simulink model "Intergration_simu"  (R2018b)
settings: Solver=FixedStepDiscrete  StartTime=0.0  StopTime=14  FixedStep=0.005  RelTol=1e-3
PostLoadFcn:
  | if any(exist('dsrtsu_mdlpostloadfcn', 'file') ~= 0), dsrtsu_mdlpostloadfcn('Execute', bdroot); end
values from neighbouring files (symbols this model uses):
  P_x165_On = 1.0    [CAN_Tx.sldd]
  P_x242_On = 1.0    [CAN_Tx.sldd]
  P_x246_On = 1.0    [CAN_Tx.sldd]
libraries: rtican x112, simulink x59
(part 29 of 31)

== system Intergration_simu/Radar410_RX/Subsystem41/Subsystem21 ==
  In1 : Inport
  Bus Creator : BusCreator  Inputs=20  OutDataTypeStr=Bus: Obj_Data  NonVirtualBus=on
      settings: InheritFromInputs=off
  Bus Selector : BusSelector  OutputSignals=FRS_P1_19_Msg_CheckSum,FRS_P1_19_Msg_AliveCounter,FRS_P1_19_Obj_ExstProb,FRS_P1_19_Obj_XVelRel_Stdev,FRS_P1_19_Obj_XAccRel,FRS_P1_19_Obj_ObstacleProb,FRS_P1_19_Obj_MotionPattern,FRS_P1_19_Obj_YPos_Stdev,FRS_P1_19_Obj_ValidFlag,FRS_P1_19_Obj_XPos_Stdev,FRS_P1_19_Obj_UpdateFlag,FRS_P1_19_Obj_ID,FRS_P2_19_Msg_CheckSum,FRS_P2_19_Msg_AliveCounter,FRS_P2_19_Obj_MeasFlag,FRS_P2_19_Obj_YVelRel,FRS_P2_19_Obj_Type,FRS_P2_19_Obj_XPos,FRS_P2_19_Obj_YPos,FRS_P2_19_Obj_XVelRel
  Data Type Conversion{,1..19} (20 alike) : DataTypeConversion  OutDataTypeStr=single
  Out1 : Outport  OutDataTypeStr=Bus: Obj_Data
  wires:
  Data Type Conversion19/1 -> Bus Creator/20
  Data Type Conversion14/1 -> Bus Creator/15
  Data Type Conversion8/1 -> Bus Creator/9
  Data Type Conversion7/1 -> Bus Creator/8
  Data Type Conversion3/1 -> Bus Creator/4
  Data Type Conversion4/1 -> Bus Creator/5
  Data Type Conversion1/1 -> Bus Creator/2
  Data Type Conversion13/1 -> Bus Creator/14
  Data Type Conversion2/1 -> Bus Creator/3
  Data Type Conversion/1 -> Bus Creator/1
  Bus Creator/1 -> Out1/1
  In1/1 -> Bus Selector/1
  Bus Selector/20 -> Data Type Conversion19/1  "<FRS_P2_19_Obj_XVelRel>"
  Bus Selector/18 -> Data Type Conversion17/1  "<FRS_P2_19_Obj_XPos>"
  Bus Selector/19 -> Data Type Conversion18/1  "<FRS_P2_19_Obj_YPos>"
  Bus Selector/14 -> Data Type Conversion13/1  "<FRS_P2_19_Msg_AliveCounter>"
  Data Type Conversion10/1 -> Bus Creator/11
  Bus Selector/10 -> Data Type Conversion9/1  "<FRS_P1_19_Obj_XPos_Stdev>"
  Bus Selector/17 -> Data Type Conversion16/1  "<FRS_P2_19_Obj_Type>"
  Bus Selector/9 -> Data Type Conversion8/1  "<FRS_P1_19_Obj_ValidFlag>"
  Data Type Conversion16/1 -> Bus Creator/17
  Bus Selector/12 -> Data Type Conversion11/1  "<FRS_P1_19_Obj_ID>"
  Data Type Conversion6/1 -> Bus Creator/7
  Bus Selector/16 -> Data Type Conversion15/1  "<FRS_P2_19_Obj_YVelRel>"
  Data Type Conversion17/1 -> Bus Creator/18
  Bus Selector/11 -> Data Type Conversion10/1  "<FRS_P1_19_Obj_UpdateFlag>"
  Data Type Conversion18/1 -> Bus Creator/19
  Bus Selector/6 -> Data Type Conversion5/1  "<FRS_P1_19_Obj_ObstacleProb>"
  Data Type Conversion9/1 -> Bus Creator/10
  Bus Selector/7 -> Data Type Conversion6/1  "<FRS_P1_19_Obj_MotionPattern>"
  Bus Selector/4 -> Data Type Conversion3/1  "<FRS_P1_19_Obj_XVelRel_Stdev>"
  Data Type Conversion5/1 -> Bus Creator/6
  Data Type Conversion11/1 -> Bus Creator/12
  Bus Selector/2 -> Data Type Conversion1/1  "<FRS_P1_19_Msg_AliveCounter>"
  Bus Selector/13 -> Data Type Conversion12/1  "<FRS_P2_19_Msg_CheckSum>"
  Bus Selector/3 -> Data Type Conversion2/1  "<FRS_P1_19_Obj_ExstProb>"
  Bus Selector/15 -> Data Type Conversion14/1  "<FRS_P2_19_Obj_MeasFlag>"
  Bus Selector/1 -> Data Type Conversion/1  "<FRS_P1_19_Msg_CheckSum>"
  Data Type Conversion15/1 -> Bus Creator/16
  Bus Selector/8 -> Data Type Conversion7/1  "<FRS_P1_19_Obj_YPos_Stdev>"
  Bus Selector/5 -> Data Type Conversion4/1  "<FRS_P1_19_Obj_XAccRel>"
  Data Type Conversion12/1 -> Bus Creator/13

== system Intergration_simu/Radar410_RX/Subsystem41/Subsystem22 ==
  In1 : Inport
  Bus Creator : BusCreator  Inputs=20  OutDataTypeStr=Bus: Obj_Data  NonVirtualBus=on
      settings: InheritFromInputs=off
  Bus Selector : BusSelector  OutputSignals=FRS_P1_20_Msg_CheckSum,FRS_P1_20_Msg_AliveCounter,FRS_P1_20_Obj_ExstProb,FRS_P1_20_Obj_XVelRel_Stdev,FRS_P1_20_Obj_XAccRel,FRS_P1_20_Obj_ObstacleProb,FRS_P1_20_Obj_MotionPattern,FRS_P1_20_Obj_YPos_Stdev,FRS_P1_20_Obj_ValidFlag,FRS_P1_20_Obj_XPos_Stdev,FRS_P1_20_Obj_UpdateFlag,FRS_P1_20_Obj_ID,FRS_P2_20_Msg_CheckSum,FRS_P2_20_Msg_AliveCounter,FRS_P2_20_Obj_MeasFlag,FRS_P2_20_Obj_YVelRel,FRS_P2_20_Obj_Type,FRS_P2_20_Obj_XPos,FRS_P2_20_Obj_YPos,FRS_P2_20_Obj_XVelRel
  Data Type Conversion{,1..19} (20 alike) : DataTypeConversion  OutDataTypeStr=single
  Out1 : Outport  OutDataTypeStr=Bus: Obj_Data
  wires:
  Data Type Conversion19/1 -> Bus Creator/20
  Data Type Conversion14/1 -> Bus Creator/15
  Data Type Conversion8/1 -> Bus Creator/9
  Data Type Conversion7/1 -> Bus Creator/8
  Data Type Conversion3/1 -> Bus Creator/4
  Data Type Conversion4/1 -> Bus Creator/5
  Data Type Conversion1/1 -> Bus Creator/2
  Data Type Conversion13/1 -> Bus Creator/14
  Data Type Conversion2/1 -> Bus Creator/3
  Data Type Conversion/1 -> Bus Creator/1
  Bus Creator/1 -> Out1/1
  In1/1 -> Bus Selector/1
  Bus Selector/20 -> Data Type Conversion19/1  "<FRS_P2_20_Obj_XVelRel>"
  Bus Selector/18 -> Data Type Conversion17/1  "<FRS_P2_20_Obj_XPos>"
  Bus Selector/19 -> Data Type Conversion18/1  "<FRS_P2_20_Obj_YPos>"
  Bus Selector/14 -> Data Type Conversion13/1  "<FRS_P2_20_Msg_AliveCounter>"
  Data Type Conversion10/1 -> Bus Creator/11
  Bus Selector/10 -> Data Type Conversion9/1  "<FRS_P1_20_Obj_XPos_Stdev>"
  Bus Selector/17 -> Data Type Conversion16/1  "<FRS_P2_20_Obj_Type>"
  Bus Selector/9 -> Data Type Conversion8/1  "<FRS_P1_20_Obj_ValidFlag>"
  Data Type Conversion16/1 -> Bus Creator/17
  Bus Selector/12 -> Data Type Conversion11/1  "<FRS_P1_20_Obj_ID>"
  Data Type Conversion6/1 -> Bus Creator/7
  Bus Selector/16 -> Data Type Conversion15/1  "<FRS_P2_20_Obj_YVelRel>"
  Data Type Conversion17/1 -> Bus Creator/18
  Bus Selector/11 -> Data Type Conversion10/1  "<FRS_P1_20_Obj_UpdateFlag>"
  Data Type Conversion18/1 -> Bus Creator/19
  Bus Selector/6 -> Data Type Conversion5/1  "<FRS_P1_20_Obj_ObstacleProb>"
  Data Type Conversion9/1 -> Bus Creator/10
  Bus Selector/7 -> Data Type Conversion6/1  "<FRS_P1_20_Obj_MotionPattern>"
  Bus Selector/4 -> Data Type Conversion3/1  "<FRS_P1_20_Obj_XVelRel_Stdev>"
  Data Type Conversion5/1 -> Bus Creator/6
  Data Type Conversion11/1 -> Bus Creator/12
  Bus Selector/2 -> Data Type Conversion1/1  "<FRS_P1_20_Msg_AliveCounter>"
  Bus Selector/13 -> Data Type Conversion12/1  "<FRS_P2_20_Msg_CheckSum>"
  Bus Selector/3 -> Data Type Conversion2/1  "<FRS_P1_20_Obj_ExstProb>"
  Bus Selector/15 -> Data Type Conversion14/1  "<FRS_P2_20_Obj_MeasFlag>"
  Bus Selector/1 -> Data Type Conversion/1  "<FRS_P1_20_Msg_CheckSum>"
  Data Type Conversion15/1 -> Bus Creator/16
  Bus Selector/8 -> Data Type Conversion7/1  "<FRS_P1_20_Obj_YPos_Stdev>"
  Bus Selector/5 -> Data Type Conversion4/1  "<FRS_P1_20_Obj_XAccRel>"
  Data Type Conversion12/1 -> Bus Creator/13

== system Intergration_simu/Radar410_RX/Subsystem41/Subsystem23 ==
  In1 : Inport
  Bus Creator : BusCreator  Inputs=20  OutDataTypeStr=Bus: Obj_Data  NonVirtualBus=on
      settings: InheritFromInputs=off
  Bus Selector : BusSelector  OutputSignals=FRS_P1_21_Msg_CheckSum,FRS_P1_21_Msg_AliveCounter,FRS_P1_21_Obj_ExstProb,FRS_P1_21_Obj_XVelRel_Stdev,FRS_P1_21_Obj_XAccRel,FRS_P1_21_Obj_ObstacleProb,FRS_P1_21_Obj_MotionPattern,FRS_P1_21_Obj_YPos_Stdev,FRS_P1_21_Obj_ValidFlag,FRS_P1_21_Obj_XPos_Stdev,FRS_P1_21_Obj_UpdateFlag,FRS_P1_21_Obj_ID,FRS_P2_21_Msg_CheckSum,FRS_P2_21_Msg_AliveCounter,FRS_P2_21_Obj_MeasFlag,FRS_P2_21_Obj_YVelRel,FRS_P2_21_Obj_Type,FRS_P2_21_Obj_XPos,FRS_P2_21_Obj_YPos,FRS_P2_21_Obj_XVelRel
  Data Type Conversion{,1..19} (20 alike) : DataTypeConversion  OutDataTypeStr=single
  Out1 : Outport  OutDataTypeStr=Bus: Obj_Data
  wires:
  Data Type Conversion12/1 -> Bus Creator/13
  Bus Selector/5 -> Data Type Conversion4/1  "<FRS_P1_21_Obj_XAccRel>"
  Bus Selector/8 -> Data Type Conversion7/1  "<FRS_P1_21_Obj_YPos_Stdev>"
  Data Type Conversion15/1 -> Bus Creator/16
  Bus Selector/1 -> Data Type Conversion/1  "<FRS_P1_21_Msg_CheckSum>"
  Bus Selector/15 -> Data Type Conversion14/1  "<FRS_P2_21_Obj_MeasFlag>"
  Bus Selector/3 -> Data Type Conversion2/1  "<FRS_P1_21_Obj_ExstProb>"
  Bus Selector/13 -> Data Type Conversion12/1  "<FRS_P2_21_Msg_CheckSum>"
  Bus Selector/2 -> Data Type Conversion1/1  "<FRS_P1_21_Msg_AliveCounter>"
  Data Type Conversion11/1 -> Bus Creator/12
  Data Type Conversion5/1 -> Bus Creator/6
  Bus Selector/4 -> Data Type Conversion3/1  "<FRS_P1_21_Obj_XVelRel_Stdev>"
  Bus Selector/7 -> Data Type Conversion6/1  "<FRS_P1_21_Obj_MotionPattern>"
  Data Type Conversion9/1 -> Bus Creator/10
  Bus Selector/6 -> Data Type Conversion5/1  "<FRS_P1_21_Obj_ObstacleProb>"
  Data Type Conversion18/1 -> Bus Creator/19
  Bus Selector/11 -> Data Type Conversion10/1  "<FRS_P1_21_Obj_UpdateFlag>"
  Data Type Conversion17/1 -> Bus Creator/18
  Bus Selector/16 -> Data Type Conversion15/1  "<FRS_P2_21_Obj_YVelRel>"
  Data Type Conversion6/1 -> Bus Creator/7
  Bus Selector/12 -> Data Type Conversion11/1  "<FRS_P1_21_Obj_ID>"
  Data Type Conversion16/1 -> Bus Creator/17
  Bus Selector/9 -> Data Type Conversion8/1  "<FRS_P1_21_Obj_ValidFlag>"
  Bus Selector/17 -> Data Type Conversion16/1  "<FRS_P2_21_Obj_Type>"
  Bus Selector/10 -> Data Type Conversion9/1  "<FRS_P1_21_Obj_XPos_Stdev>"
  Data Type Conversion10/1 -> Bus Creator/11
  Bus Selector/14 -> Data Type Conversion13/1  "<FRS_P2_21_Msg_AliveCounter>"
  Bus Selector/19 -> Data Type Conversion18/1  "<FRS_P2_21_Obj_YPos>"
  Bus Selector/18 -> Data Type Conversion17/1  "<FRS_P2_21_Obj_XPos>"
  Bus Selector/20 -> Data Type Conversion19/1  "<FRS_P2_21_Obj_XVelRel>"
  In1/1 -> Bus Selector/1
  Bus Creator/1 -> Out1/1
  Data Type Conversion/1 -> Bus Creator/1
  Data Type Conversion2/1 -> Bus Creator/3
  Data Type Conversion13/1 -> Bus Creator/14
  Data Type Conversion1/1 -> Bus Creator/2
  Data Type Conversion4/1 -> Bus Creator/5
  Data Type Conversion3/1 -> Bus Creator/4
  Data Type Conversion7/1 -> Bus Creator/8
  Data Type Conversion8/1 -> Bus Creator/9
  Data Type Conversion14/1 -> Bus Creator/15
  Data Type Conversion19/1 -> Bus Creator/20

== system Intergration_simu/Radar410_RX/Subsystem41/Subsystem24 ==
  In1 : Inport
  Bus Creator : BusCreator  Inputs=20  OutDataTypeStr=Bus: Obj_Data  NonVirtualBus=on
      settings: InheritFromInputs=off
  Bus Selector : BusSelector  OutputSignals=FRS_P1_24_Msg_CheckSum,FRS_P1_24_Msg_AliveCounter,FRS_P1_24_Obj_ExstProb,FRS_P1_24_Obj_XVelRel_Stdev,FRS_P1_24_Obj_XAccRel,FRS_P1_24_Obj_ObstacleProb,FRS_P1_24_Obj_MotionPattern,FRS_P1_24_Obj_YPos_Stdev,FRS_P1_24_Obj_ValidFlag,FRS_P1_24_Obj_XPos_Stdev,FRS_P1_24_Obj_UpdateFlag,FRS_P1_24_Obj_ID,FRS_P2_24_Msg_CheckSum,FRS_P2_24_Msg_AliveCounter,FRS_P2_24_Obj_MeasFlag,FRS_P2_24_Obj_YVelRel,FRS_P2_24_Obj_Type,FRS_P2_24_Obj_XPos,FRS_P2_24_Obj_YPos,FRS_P2_24_Obj_XVelRel
  Data Type Conversion{,1..19} (20 alike) : DataTypeConversion  OutDataTypeStr=single
  Out1 : Outport  OutDataTypeStr=Bus: Obj_Data
  wires:
  Data Type Conversion12/1 -> Bus Creator/13
  Bus Selector/5 -> Data Type Conversion4/1  "<FRS_P1_24_Obj_XAccRel>"
  Bus Selector/8 -> Data Type Conversion7/1  "<FRS_P1_24_Obj_YPos_Stdev>"
  Data Type Conversion15/1 -> Bus Creator/16
  Bus Selector/1 -> Data Type Conversion/1  "<FRS_P1_24_Msg_CheckSum>"
  Bus Selector/15 -> Data Type Conversion14/1  "<FRS_P2_24_Obj_MeasFlag>"
  Bus Selector/3 -> Data Type Conversion2/1  "<FRS_P1_24_Obj_ExstProb>"
  Bus Selector/13 -> Data Type Conversion12/1  "<FRS_P2_24_Msg_CheckSum>"
  Bus Selector/2 -> Data Type Conversion1/1  "<FRS_P1_24_Msg_AliveCounter>"
  Data Type Conversion11/1 -> Bus Creator/12
  Data Type Conversion5/1 -> Bus Creator/6
  Bus Selector/4 -> Data Type Conversion3/1  "<FRS_P1_24_Obj_XVelRel_Stdev>"
  Bus Selector/7 -> Data Type Conversion6/1  "<FRS_P1_24_Obj_MotionPattern>"
  Data Type Conversion9/1 -> Bus Creator/10
  Bus Selector/6 -> Data Type Conversion5/1  "<FRS_P1_24_Obj_ObstacleProb>"
  Data Type Conversion18/1 -> Bus Creator/19
  Bus Selector/11 -> Data Type Conversion10/1  "<FRS_P1_24_Obj_UpdateFlag>"
  Data Type Conversion17/1 -> Bus Creator/18
  Bus Selector/16 -> Data Type Conversion15/1  "<FRS_P2_24_Obj_YVelRel>"
  Data Type Conversion6/1 -> Bus Creator/7
  Bus Selector/12 -> Data Type Conversion11/1  "<FRS_P1_24_Obj_ID>"
  Data Type Conversion16/1 -> Bus Creator/17
  Bus Selector/9 -> Data Type Conversion8/1  "<FRS_P1_24_Obj_ValidFlag>"
  Bus Selector/17 -> Data Type Conversion16/1  "<FRS_P2_24_Obj_Type>"
  Bus Selector/10 -> Data Type Conversion9/1  "<FRS_P1_24_Obj_XPos_Stdev>"
  Data Type Conversion10/1 -> Bus Creator/11
  Bus Selector/14 -> Data Type Conversion13/1  "<FRS_P2_24_Msg_AliveCounter>"
  Bus Selector/19 -> Data Type Conversion18/1  "<FRS_P2_24_Obj_YPos>"
  Bus Selector/18 -> Data Type Conversion17/1  "<FRS_P2_24_Obj_XPos>"
  Bus Selector/20 -> Data Type Conversion19/1  "<FRS_P2_24_Obj_XVelRel>"
  In1/1 -> Bus Selector/1
  Bus Creator/1 -> Out1/1
  Data Type Conversion/1 -> Bus Creator/1
  Data Type Conversion2/1 -> Bus Creator/3
  Data Type Conversion13/1 -> Bus Creator/14
  Data Type Conversion1/1 -> Bus Creator/2
  Data Type Conversion4/1 -> Bus Creator/5
  Data Type Conversion3/1 -> Bus Creator/4
  Data Type Conversion7/1 -> Bus Creator/8
  Data Type Conversion8/1 -> Bus Creator/9
  Data Type Conversion14/1 -> Bus Creator/15
  Data Type Conversion19/1 -> Bus Creator/20

== system Intergration_simu/Radar410_RX/Subsystem41/Subsystem25 ==
  In1 : Inport
  Bus Creator : BusCreator  Inputs=20  OutDataTypeStr=Bus: Obj_Data  NonVirtualBus=on
      settings: InheritFromInputs=off
  Bus Selector : BusSelector  OutputSignals=FRS_P1_25_Msg_CheckSum,FRS_P1_25_Msg_AliveCounter,FRS_P1_25_Obj_ExstProb,FRS_P1_25_Obj_XVelRel_Stdev,FRS_P1_25_Obj_XAccRel,FRS_P1_25_Obj_ObstacleProb,FRS_P1_25_Obj_MotionPattern,FRS_P1_25_Obj_YPos_Stdev,FRS_P1_25_Obj_ValidFlag,FRS_P1_25_Obj_XPos_Stdev,FRS_P1_25_Obj_UpdateFlag,FRS_P1_25_Obj_ID,FRS_P2_25_Msg_CheckSum,FRS_P2_25_Msg_AliveCounter,FRS_P2_25_Obj_MeasFlag,FRS_P2_25_Obj_YVelRel,FRS_P2_25_Obj_Type,FRS_P2_25_Obj_XPos,FRS_P2_25_Obj_YPos,FRS_P2_25_Obj_XVelRel
  Data Type Conversion{,1..19} (20 alike) : DataTypeConversion  OutDataTypeStr=single
  Out1 : Outport  OutDataTypeStr=Bus: Obj_Data
  wires:
  Data Type Conversion19/1 -> Bus Creator/20
  Data Type Conversion14/1 -> Bus Creator/15
  Data Type Conversion8/1 -> Bus Creator/9
  Data Type Conversion7/1 -> Bus Creator/8
  Data Type Conversion3/1 -> Bus Creator/4
  Data Type Conversion4/1 -> Bus Creator/5
  Data Type Conversion1/1 -> Bus Creator/2
  Data Type Conversion13/1 -> Bus Creator/14
  Data Type Conversion2/1 -> Bus Creator/3
  Data Type Conversion/1 -> Bus Creator/1
  Bus Creator/1 -> Out1/1
  In1/1 -> Bus Selector/1
  Bus Selector/20 -> Data Type Conversion19/1  "<FRS_P2_25_Obj_XVelRel>"
  Bus Selector/18 -> Data Type Conversion17/1  "<FRS_P2_25_Obj_XPos>"
  Bus Selector/19 -> Data Type Conversion18/1  "<FRS_P2_25_Obj_YPos>"
  Bus Selector/14 -> Data Type Conversion13/1  "<FRS_P2_25_Msg_AliveCounter>"
  Data Type Conversion10/1 -> Bus Creator/11
  Bus Selector/10 -> Data Type Conversion9/1  "<FRS_P1_25_Obj_XPos_Stdev>"
  Bus Selector/17 -> Data Type Conversion16/1  "<FRS_P2_25_Obj_Type>"
  Bus Selector/9 -> Data Type Conversion8/1  "<FRS_P1_25_Obj_ValidFlag>"
  Data Type Conversion16/1 -> Bus Creator/17
  Bus Selector/12 -> Data Type Conversion11/1  "<FRS_P1_25_Obj_ID>"
  Data Type Conversion6/1 -> Bus Creator/7
  Bus Selector/16 -> Data Type Conversion15/1  "<FRS_P2_25_Obj_YVelRel>"
  Data Type Conversion17/1 -> Bus Creator/18
  Bus Selector/11 -> Data Type Conversion10/1  "<FRS_P1_25_Obj_UpdateFlag>"
  Data Type Conversion18/1 -> Bus Creator/19
  Bus Selector/6 -> Data Type Conversion5/1  "<FRS_P1_25_Obj_ObstacleProb>"
  Data Type Conversion9/1 -> Bus Creator/10
  Bus Selector/7 -> Data Type Conversion6/1  "<FRS_P1_25_Obj_MotionPattern>"
  Bus Selector/4 -> Data Type Conversion3/1  "<FRS_P1_25_Obj_XVelRel_Stdev>"
  Data Type Conversion5/1 -> Bus Creator/6
  Data Type Conversion11/1 -> Bus Creator/12
  Bus Selector/2 -> Data Type Conversion1/1  "<FRS_P1_25_Msg_AliveCounter>"
  Bus Selector/13 -> Data Type Conversion12/1  "<FRS_P2_25_Msg_CheckSum>"
  Bus Selector/3 -> Data Type Conversion2/1  "<FRS_P1_25_Obj_ExstProb>"
  Bus Selector/15 -> Data Type Conversion14/1  "<FRS_P2_25_Obj_MeasFlag>"
  Bus Selector/1 -> Data Type Conversion/1  "<FRS_P1_25_Msg_CheckSum>"
  Data Type Conversion15/1 -> Bus Creator/16
  Bus Selector/8 -> Data Type Conversion7/1  "<FRS_P1_25_Obj_YPos_Stdev>"
  Bus Selector/5 -> Data Type Conversion4/1  "<FRS_P1_25_Obj_XAccRel>"
  Data Type Conversion12/1 -> Bus Creator/13

== system Intergration_simu/Radar410_RX/Subsystem41/Subsystem26 ==
  In1 : Inport
  Bus Creator : BusCreator  Inputs=20  OutDataTypeStr=Bus: Obj_Data  NonVirtualBus=on
      settings: InheritFromInputs=off
  Bus Selector : BusSelector  OutputSignals=FRS_P1_34_Msg_CheckSum,FRS_P1_34_Msg_AliveCounter,FRS_P1_34_Obj_ExstProb,FRS_P1_34_Obj_XVelRel_Stdev,FRS_P1_34_Obj_XAccRel,FRS_P1_34_Obj_ObstacleProb,FRS_P1_34_Obj_MotionPattern,FRS_P1_34_Obj_YPos_Stdev,FRS_P1_34_Obj_ValidFlag,FRS_P1_34_Obj_XPos_Stdev,FRS_P1_34_Obj_UpdateFlag,FRS_P1_34_Obj_ID,FRS_P2_34_Msg_CheckSum,FRS_P2_34_Msg_AliveCounter,FRS_P2_34_Obj_MeasFlag,FRS_P2_34_Obj_YVelRel,FRS_P2_34_Obj_Type,FRS_P2_34_Obj_XPos,FRS_P2_34_Obj_YPos,FRS_P2_34_Obj_XVelRel
  Data Type Conversion{,1..19} (20 alike) : DataTypeConversion  OutDataTypeStr=single
  Out1 : Outport  OutDataTypeStr=Bus: Obj_Data
  wires:
  Data Type Conversion19/1 -> Bus Creator/20
  Data Type Conversion14/1 -> Bus Creator/15
  Data Type Conversion8/1 -> Bus Creator/9
  Data Type Conversion7/1 -> Bus Creator/8
  Data Type Conversion3/1 -> Bus Creator/4
  Data Type Conversion4/1 -> Bus Creator/5
  Data Type Conversion1/1 -> Bus Creator/2
  Data Type Conversion13/1 -> Bus Creator/14
  Data Type Conversion2/1 -> Bus Creator/3
  Data Type Conversion/1 -> Bus Creator/1
  Bus Creator/1 -> Out1/1
  In1/1 -> Bus Selector/1
  Bus Selector/20 -> Data Type Conversion19/1  "<FRS_P2_34_Obj_XVelRel>"
  Bus Selector/18 -> Data Type Conversion17/1  "<FRS_P2_34_Obj_XPos>"
  Bus Selector/19 -> Data Type Conversion18/1  "<FRS_P2_34_Obj_YPos>"
  Bus Selector/14 -> Data Type Conversion13/1  "<FRS_P2_34_Msg_AliveCounter>"
  Data Type Conversion10/1 -> Bus Creator/11
  Bus Selector/10 -> Data Type Conversion9/1  "<FRS_P1_34_Obj_XPos_Stdev>"
  Bus Selector/17 -> Data Type Conversion16/1  "<FRS_P2_34_Obj_Type>"
  Bus Selector/9 -> Data Type Conversion8/1  "<FRS_P1_34_Obj_ValidFlag>"
  Data Type Conversion16/1 -> Bus Creator/17
  Bus Selector/12 -> Data Type Conversion11/1  "<FRS_P1_34_Obj_ID>"
  Data Type Conversion6/1 -> Bus Creator/7
  Bus Selector/16 -> Data Type Conversion15/1  "<FRS_P2_34_Obj_YVelRel>"
  Data Type Conversion17/1 -> Bus Creator/18
  Bus Selector/11 -> Data Type Conversion10/1  "<FRS_P1_34_Obj_UpdateFlag>"
  Data Type Conversion18/1 -> Bus Creator/19
  Bus Selector/6 -> Data Type Conversion5/1  "<FRS_P1_34_Obj_ObstacleProb>"
  Data Type Conversion9/1 -> Bus Creator/10
  Bus Selector/7 -> Data Type Conversion6/1  "<FRS_P1_34_Obj_MotionPattern>"
  Bus Selector/4 -> Data Type Conversion3/1  "<FRS_P1_34_Obj_XVelRel_Stdev>"
  Data Type Conversion5/1 -> Bus Creator/6
  Data Type Conversion11/1 -> Bus Creator/12
  Bus Selector/2 -> Data Type Conversion1/1  "<FRS_P1_34_Msg_AliveCounter>"
  Bus Selector/13 -> Data Type Conversion12/1  "<FRS_P2_34_Msg_CheckSum>"
  Bus Selector/3 -> Data Type Conversion2/1  "<FRS_P1_34_Obj_ExstProb>"
  Bus Selector/15 -> Data Type Conversion14/1  "<FRS_P2_34_Obj_MeasFlag>"
  Bus Selector/1 -> Data Type Conversion/1  "<FRS_P1_34_Msg_CheckSum>"
  Data Type Conversion15/1 -> Bus Creator/16
  Bus Selector/8 -> Data Type Conversion7/1  "<FRS_P1_34_Obj_YPos_Stdev>"
  Bus Selector/5 -> Data Type Conversion4/1  "<FRS_P1_34_Obj_XAccRel>"
  Data Type Conversion12/1 -> Bus Creator/13

== system Intergration_simu/Radar410_RX/Subsystem41/Subsystem27 ==
  In1 : Inport
  Bus Creator : BusCreator  Inputs=20  OutDataTypeStr=Bus: Obj_Data  NonVirtualBus=on
      settings: InheritFromInputs=off
  Bus Selector : BusSelector  OutputSignals=FRS_P1_35_Msg_CheckSum,FRS_P1_35_Msg_AliveCounter,FRS_P1_35_Obj_ExstProb,FRS_P1_35_Obj_XVelRel_Stdev,FRS_P1_35_Obj_XAccRel,FRS_P1_35_Obj_ObstacleProb,FRS_P1_35_Obj_MotionPattern,FRS_P1_35_Obj_YPos_Stdev,FRS_P1_35_Obj_ValidFlag,FRS_P1_35_Obj_XPos_Stdev,FRS_P1_35_Obj_UpdateFlag,FRS_P1_35_Obj_ID,FRS_P2_35_Msg_CheckSum,FRS_P2_35_Msg_AliveCounter,FRS_P2_35_Obj_MeasFlag,FRS_P2_35_Obj_YVelRel,FRS_P2_35_Obj_Type,FRS_P2_35_Obj_XPos,FRS_P2_35_Obj_YPos,FRS_P2_35_Obj_XVelRel
  Data Type Conversion{,1..19} (20 alike) : DataTypeConversion  OutDataTypeStr=single
  Out1 : Outport  OutDataTypeStr=Bus: Obj_Data
  wires:
  Data Type Conversion12/1 -> Bus Creator/13
  Bus Selector/5 -> Data Type Conversion4/1  "<FRS_P1_35_Obj_XAccRel>"
  Bus Selector/8 -> Data Type Conversion7/1  "<FRS_P1_35_Obj_YPos_Stdev>"
  Data Type Conversion15/1 -> Bus Creator/16
  Bus Selector/1 -> Data Type Conversion/1  "<FRS_P1_35_Msg_CheckSum>"
  Bus Selector/15 -> Data Type Conversion14/1  "<FRS_P2_35_Obj_MeasFlag>"
  Bus Selector/3 -> Data Type Conversion2/1  "<FRS_P1_35_Obj_ExstProb>"
  Bus Selector/13 -> Data Type Conversion12/1  "<FRS_P2_35_Msg_CheckSum>"
  Bus Selector/2 -> Data Type Conversion1/1  "<FRS_P1_35_Msg_AliveCounter>"
  Data Type Conversion11/1 -> Bus Creator/12
  Data Type Conversion5/1 -> Bus Creator/6
  Bus Selector/4 -> Data Type Conversion3/1  "<FRS_P1_35_Obj_XVelRel_Stdev>"
  Bus Selector/7 -> Data Type Conversion6/1  "<FRS_P1_35_Obj_MotionPattern>"
  Data Type Conversion9/1 -> Bus Creator/10
  Bus Selector/6 -> Data Type Conversion5/1  "<FRS_P1_35_Obj_ObstacleProb>"
  Data Type Conversion18/1 -> Bus Creator/19
  Bus Selector/11 -> Data Type Conversion10/1  "<FRS_P1_35_Obj_UpdateFlag>"
  Data Type Conversion17/1 -> Bus Creator/18
  Bus Selector/16 -> Data Type Conversion15/1  "<FRS_P2_35_Obj_YVelRel>"
  Data Type Conversion6/1 -> Bus Creator/7
  Bus Selector/12 -> Data Type Conversion11/1  "<FRS_P1_35_Obj_ID>"
  Data Type Conversion16/1 -> Bus Creator/17
  Bus Selector/9 -> Data Type Conversion8/1  "<FRS_P1_35_Obj_ValidFlag>"
  Bus Selector/17 -> Data Type Conversion16/1  "<FRS_P2_35_Obj_Type>"
  Bus Selector/10 -> Data Type Conversion9/1  "<FRS_P1_35_Obj_XPos_Stdev>"
  Data Type Conversion10/1 -> Bus Creator/11
  Bus Selector/14 -> Data Type Conversion13/1  "<FRS_P2_35_Msg_AliveCounter>"
  Bus Selector/19 -> Data Type Conversion18/1  "<FRS_P2_35_Obj_YPos>"
  Bus Selector/18 -> Data Type Conversion17/1  "<FRS_P2_35_Obj_XPos>"
  Bus Selector/20 -> Data Type Conversion19/1  "<FRS_P2_35_Obj_XVelRel>"
  In1/1 -> Bus Selector/1
  Bus Creator/1 -> Out1/1
  Data Type Conversion/1 -> Bus Creator/1
  Data Type Conversion2/1 -> Bus Creator/3
  Data Type Conversion13/1 -> Bus Creator/14
  Data Type Conversion1/1 -> Bus Creator/2
  Data Type Conversion4/1 -> Bus Creator/5
  Data Type Conversion3/1 -> Bus Creator/4
  Data Type Conversion7/1 -> Bus Creator/8
  Data Type Conversion8/1 -> Bus Creator/9
  Data Type Conversion14/1 -> Bus Creator/15
  Data Type Conversion19/1 -> Bus Creator/20

== system Intergration_simu/Radar410_RX/Subsystem41/Subsystem28 ==
  In1 : Inport
  Bus Creator : BusCreator  Inputs=20  OutDataTypeStr=Bus: Obj_Data  NonVirtualBus=on
      settings: InheritFromInputs=off
  Bus Selector : BusSelector  OutputSignals=FRS_P1_26_Msg_CheckSum,FRS_P1_26_Msg_AliveCounter,FRS_P1_26_Obj_ExstProb,FRS_P1_26_Obj_XVelRel_Stdev,FRS_P1_26_Obj_XAccRel,FRS_P1_26_Obj_ObstacleProb,FRS_P1_26_Obj_MotionPattern,FRS_P1_26_Obj_YPos_Stdev,FRS_P1_26_Obj_ValidFlag,FRS_P1_26_Obj_XPos_Stdev,FRS_P1_26_Obj_UpdateFlag,FRS_P1_26_Obj_ID,FRS_P2_26_Msg_CheckSum,FRS_P2_26_Msg_AliveCounter,FRS_P2_26_Obj_MeasFlag,FRS_P2_26_Obj_YVelRel,FRS_P2_26_Obj_Type,FRS_P2_26_Obj_XPos,FRS_P2_26_Obj_YPos,FRS_P2_26_Obj_XVelRel
  Data Type Conversion{,1..19} (20 alike) : DataTypeConversion  OutDataTypeStr=single
  Out1 : Outport  OutDataTypeStr=Bus: Obj_Data
  wires:
  Data Type Conversion19/1 -> Bus Creator/20
  Data Type Conversion14/1 -> Bus Creator/15
  Data Type Conversion8/1 -> Bus Creator/9
  Data Type Conversion7/1 -> Bus Creator/8
  Data Type Conversion3/1 -> Bus Creator/4
  Data Type Conversion4/1 -> Bus Creator/5
  Data Type Conversion1/1 -> Bus Creator/2
  Data Type Conversion13/1 -> Bus Creator/14
  Data Type Conversion2/1 -> Bus Creator/3
  Data Type Conversion/1 -> Bus Creator/1
  Bus Creator/1 -> Out1/1
  In1/1 -> Bus Selector/1
  Bus Selector/20 -> Data Type Conversion19/1  "<FRS_P2_26_Obj_XVelRel>"
  Bus Selector/18 -> Data Type Conversion17/1  "<FRS_P2_26_Obj_XPos>"
  Bus Selector/19 -> Data Type Conversion18/1  "<FRS_P2_26_Obj_YPos>"
  Bus Selector/14 -> Data Type Conversion13/1  "<FRS_P2_26_Msg_AliveCounter>"
  Data Type Conversion10/1 -> Bus Creator/11
  Bus Selector/10 -> Data Type Conversion9/1  "<FRS_P1_26_Obj_XPos_Stdev>"
  Bus Selector/17 -> Data Type Conversion16/1  "<FRS_P2_26_Obj_Type>"
  Bus Selector/9 -> Data Type Conversion8/1  "<FRS_P1_26_Obj_ValidFlag>"
  Data Type Conversion16/1 -> Bus Creator/17
  Bus Selector/12 -> Data Type Conversion11/1  "<FRS_P1_26_Obj_ID>"
  Data Type Conversion6/1 -> Bus Creator/7
  Bus Selector/16 -> Data Type Conversion15/1  "<FRS_P2_26_Obj_YVelRel>"
  Data Type Conversion17/1 -> Bus Creator/18
  Bus Selector/11 -> Data Type Conversion10/1  "<FRS_P1_26_Obj_UpdateFlag>"
  Data Type Conversion18/1 -> Bus Creator/19
  Bus Selector/6 -> Data Type Conversion5/1  "<FRS_P1_26_Obj_ObstacleProb>"
  Data Type Conversion9/1 -> Bus Creator/10
  Bus Selector/7 -> Data Type Conversion6/1  "<FRS_P1_26_Obj_MotionPattern>"
  Bus Selector/4 -> Data Type Conversion3/1  "<FRS_P1_26_Obj_XVelRel_Stdev>"
  Data Type Conversion5/1 -> Bus Creator/6
  Data Type Conversion11/1 -> Bus Creator/12
  Bus Selector/2 -> Data Type Conversion1/1  "<FRS_P1_26_Msg_AliveCounter>"
  Bus Selector/13 -> Data Type Conversion12/1  "<FRS_P2_26_Msg_CheckSum>"
  Bus Selector/3 -> Data Type Conversion2/1  "<FRS_P1_26_Obj_ExstProb>"
  Bus Selector/15 -> Data Type Conversion14/1  "<FRS_P2_26_Obj_MeasFlag>"
  Bus Selector/1 -> Data Type Conversion/1  "<FRS_P1_26_Msg_CheckSum>"
  Data Type Conversion15/1 -> Bus Creator/16
  Bus Selector/8 -> Data Type Conversion7/1  "<FRS_P1_26_Obj_YPos_Stdev>"
  Bus Selector/5 -> Data Type Conversion4/1  "<FRS_P1_26_Obj_XAccRel>"
  Data Type Conversion12/1 -> Bus Creator/13

== system Intergration_simu/Radar410_RX/Subsystem41/Subsystem29 ==
  In1 : Inport
  Bus Creator : BusCreator  Inputs=20  OutDataTypeStr=Bus: Obj_Data  NonVirtualBus=on
      settings: InheritFromInputs=off
  Bus Selector : BusSelector  OutputSignals=FRS_P1_27_Msg_CheckSum,FRS_P1_27_Msg_AliveCounter,FRS_P1_27_Obj_ExstProb,FRS_P1_27_Obj_XVelRel_Stdev,FRS_P1_27_Obj_XAccRel,FRS_P1_27_Obj_ObstacleProb,FRS_P1_27_Obj_MotionPattern,FRS_P1_27_Obj_YPos_Stdev,FRS_P1_27_Obj_ValidFlag,FRS_P1_27_Obj_XPos_Stdev,FRS_P1_27_Obj_UpdateFlag,FRS_P1_27_Obj_ID,FRS_P2_27_Msg_CheckSum,FRS_P2_27_Msg_AliveCounter,FRS_P2_27_Obj_MeasFlag,FRS_P2_27_Obj_YVelRel,FRS_P2_27_Obj_Type,FRS_P2_27_Obj_XPos,FRS_P2_27_Obj_YPos,FRS_P2_27_Obj_XVelRel
  Data Type Conversion{,1..19} (20 alike) : DataTypeConversion  OutDataTypeStr=single
  Out1 : Outport  OutDataTypeStr=Bus: Obj_Data
  wires:
  Data Type Conversion12/1 -> Bus Creator/13
  Bus Selector/5 -> Data Type Conversion4/1  "<FRS_P1_27_Obj_XAccRel>"
  Bus Selector/8 -> Data Type Conversion7/1  "<FRS_P1_27_Obj_YPos_Stdev>"
  Data Type Conversion15/1 -> Bus Creator/16
  Bus Selector/1 -> Data Type Conversion/1  "<FRS_P1_27_Msg_CheckSum>"
  Bus Selector/15 -> Data Type Conversion14/1  "<FRS_P2_27_Obj_MeasFlag>"
  Bus Selector/3 -> Data Type Conversion2/1  "<FRS_P1_27_Obj_ExstProb>"
  Bus Selector/13 -> Data Type Conversion12/1  "<FRS_P2_27_Msg_CheckSum>"
  Bus Selector/2 -> Data Type Conversion1/1  "<FRS_P1_27_Msg_AliveCounter>"
  Data Type Conversion11/1 -> Bus Creator/12
  Data Type Conversion5/1 -> Bus Creator/6
  Bus Selector/4 -> Data Type Conversion3/1  "<FRS_P1_27_Obj_XVelRel_Stdev>"
  Bus Selector/7 -> Data Type Conversion6/1  "<FRS_P1_27_Obj_MotionPattern>"
  Data Type Conversion9/1 -> Bus Creator/10
  Bus Selector/6 -> Data Type Conversion5/1  "<FRS_P1_27_Obj_ObstacleProb>"
  Data Type Conversion18/1 -> Bus Creator/19
  Bus Selector/11 -> Data Type Conversion10/1  "<FRS_P1_27_Obj_UpdateFlag>"
  Data Type Conversion17/1 -> Bus Creator/18
  Bus Selector/16 -> Data Type Conversion15/1  "<FRS_P2_27_Obj_YVelRel>"
  Data Type Conversion6/1 -> Bus Creator/7
  Bus Selector/12 -> Data Type Conversion11/1  "<FRS_P1_27_Obj_ID>"
  Data Type Conversion16/1 -> Bus Creator/17
  Bus Selector/9 -> Data Type Conversion8/1  "<FRS_P1_27_Obj_ValidFlag>"
  Bus Selector/17 -> Data Type Conversion16/1  "<FRS_P2_27_Obj_Type>"
  Bus Selector/10 -> Data Type Conversion9/1  "<FRS_P1_27_Obj_XPos_Stdev>"
  Data Type Conversion10/1 -> Bus Creator/11
  Bus Selector/14 -> Data Type Conversion13/1  "<FRS_P2_27_Msg_AliveCounter>"
  Bus Selector/19 -> Data Type Conversion18/1  "<FRS_P2_27_Obj_YPos>"
  Bus Selector/18 -> Data Type Conversion17/1  "<FRS_P2_27_Obj_XPos>"
  Bus Selector/20 -> Data Type Conversion19/1  "<FRS_P2_27_Obj_XVelRel>"
  In1/1 -> Bus Selector/1
  Bus Creator/1 -> Out1/1
  Data Type Conversion/1 -> Bus Creator/1
  Data Type Conversion2/1 -> Bus Creator/3
  Data Type Conversion13/1 -> Bus Creator/14
  Data Type Conversion1/1 -> Bus Creator/2
  Data Type Conversion4/1 -> Bus Creator/5
  Data Type Conversion3/1 -> Bus Creator/4
  Data Type Conversion7/1 -> Bus Creator/8
  Data Type Conversion8/1 -> Bus Creator/9
  Data Type Conversion14/1 -> Bus Creator/15
  Data Type Conversion19/1 -> Bus Creator/20

== system Intergration_simu/Radar410_RX/Subsystem41/Subsystem3 ==
  In1 : Inport
  Bus Creator : BusCreator  Inputs=20  OutDataTypeStr=Bus: Obj_Data  NonVirtualBus=on
      settings: InheritFromInputs=off
  Bus Selector : BusSelector  OutputSignals=FRS_P1_03_Msg_CheckSum,FRS_P1_03_Msg_AliveCounter,FRS_P1_03_Obj_ExstProb,FRS_P1_03_Obj_XVelRel_Stdev,FRS_P1_03_Obj_XAccRel,FRS_P1_03_Obj_ObstacleProb,FRS_P1_03_Obj_MotionPattern,FRS_P1_03_Obj_YPos_Stdev,FRS_P1_03_Obj_ValidFlag,FRS_P1_03_Obj_XPos_Stdev,FRS_P1_03_Obj_UpdateFlag,FRS_P1_03_Obj_ID,FRS_P2_03_Msg_CheckSum,FRS_P2_03_Msg_AliveCounter,FRS_P2_03_Obj_MeasFlag,FRS_P2_03_Obj_YVelRel,FRS_P2_03_Obj_Type,FRS_P2_03_Obj_XPos,FRS_P2_03_Obj_YPos,FRS_P2_03_Obj_XVelRel
  Data Type Conversion{,1..19} (20 alike) : DataTypeConversion  OutDataTypeStr=single
  Out1 : Outport  OutDataTypeStr=Bus: Obj_Data
  wires:
  Data Type Conversion12/1 -> Bus Creator/13
  Bus Selector/5 -> Data Type Conversion4/1  "<FRS_P1_03_Obj_XAccRel>"
  Bus Selector/8 -> Data Type Conversion7/1  "<FRS_P1_03_Obj_YPos_Stdev>"
  Data Type Conversion15/1 -> Bus Creator/16
  Bus Selector/1 -> Data Type Conversion/1  "<FRS_P1_03_Msg_CheckSum>"
  Bus Selector/15 -> Data Type Conversion14/1  "<FRS_P2_03_Obj_MeasFlag>"
  Bus Selector/3 -> Data Type Conversion2/1  "<FRS_P1_03_Obj_ExstProb>"
  Bus Selector/13 -> Data Type Conversion12/1  "<FRS_P2_03_Msg_CheckSum>"
  Bus Selector/2 -> Data Type Conversion1/1  "<FRS_P1_03_Msg_AliveCounter>"
  Data Type Conversion11/1 -> Bus Creator/12
  Data Type Conversion5/1 -> Bus Creator/6
  Bus Selector/4 -> Data Type Conversion3/1  "<FRS_P1_03_Obj_XVelRel_Stdev>"
  Bus Selector/7 -> Data Type Conversion6/1  "<FRS_P1_03_Obj_MotionPattern>"
  Data Type Conversion9/1 -> Bus Creator/10
  Bus Selector/6 -> Data Type Conversion5/1  "<FRS_P1_03_Obj_ObstacleProb>"
  Data Type Conversion18/1 -> Bus Creator/19
  Bus Selector/11 -> Data Type Conversion10/1  "<FRS_P1_03_Obj_UpdateFlag>"
  Data Type Conversion17/1 -> Bus Creator/18
  Bus Selector/16 -> Data Type Conversion15/1  "<FRS_P2_03_Obj_YVelRel>"
  Data Type Conversion6/1 -> Bus Creator/7
  Bus Selector/12 -> Data Type Conversion11/1  "<FRS_P1_03_Obj_ID>"
  Data Type Conversion16/1 -> Bus Creator/17
  Bus Selector/9 -> Data Type Conversion8/1  "<FRS_P1_03_Obj_ValidFlag>"
  Bus Selector/17 -> Data Type Conversion16/1  "<FRS_P2_03_Obj_Type>"
  Bus Selector/10 -> Data Type Conversion9/1  "<FRS_P1_03_Obj_XPos_Stdev>"
  Data Type Conversion10/1 -> Bus Creator/11
  Bus Selector/14 -> Data Type Conversion13/1  "<FRS_P2_03_Msg_AliveCounter>"
  Bus Selector/19 -> Data Type Conversion18/1  "<FRS_P2_03_Obj_YPos>"
  Bus Selector/18 -> Data Type Conversion17/1  "<FRS_P2_03_Obj_XPos>"
  Bus Selector/20 -> Data Type Conversion19/1  "<FRS_P2_03_Obj_XVelRel>"
  In1/1 -> Bus Selector/1
  Bus Creator/1 -> Out1/1
  Data Type Conversion/1 -> Bus Creator/1
  Data Type Conversion2/1 -> Bus Creator/3
  Data Type Conversion13/1 -> Bus Creator/14
  Data Type Conversion1/1 -> Bus Creator/2
  Data Type Conversion4/1 -> Bus Creator/5
  Data Type Conversion3/1 -> Bus Creator/4
  Data Type Conversion7/1 -> Bus Creator/8
  Data Type Conversion8/1 -> Bus Creator/9
  Data Type Conversion14/1 -> Bus Creator/15
  Data Type Conversion19/1 -> Bus Creator/20

== system Intergration_simu/Radar410_RX/Subsystem41/Subsystem30 ==
  In1 : Inport
  Bus Creator : BusCreator  Inputs=20  OutDataTypeStr=Bus: Obj_Data  NonVirtualBus=on
      settings: InheritFromInputs=off
  Bus Selector : BusSelector  OutputSignals=FRS_P1_28_Msg_CheckSum,FRS_P1_28_Msg_AliveCounter,FRS_P1_28_Obj_ExstProb,FRS_P1_28_Obj_XVelRel_Stdev,FRS_P1_28_Obj_XAccRel,FRS_P1_28_Obj_ObstacleProb,FRS_P1_28_Obj_MotionPattern,FRS_P1_28_Obj_YPos_Stdev,FRS_P1_28_Obj_ValidFlag,FRS_P1_28_Obj_XPos_Stdev,FRS_P1_28_Obj_UpdateFlag,FRS_P1_28_Obj_ID,FRS_P2_28_Msg_CheckSum,FRS_P2_28_Msg_AliveCounter,FRS_P2_28_Obj_MeasFlag,FRS_P2_28_Obj_YVelRel,FRS_P2_28_Obj_Type,FRS_P2_28_Obj_XPos,FRS_P2_28_Obj_YPos,FRS_P2_28_Obj_XVelRel
  Data Type Conversion{,1..19} (20 alike) : DataTypeConversion  OutDataTypeStr=single
  Out1 : Outport  OutDataTypeStr=Bus: Obj_Data
  wires:
  Data Type Conversion12/1 -> Bus Creator/13
  Bus Selector/5 -> Data Type Conversion4/1  "<FRS_P1_28_Obj_XAccRel>"
  Bus Selector/8 -> Data Type Conversion7/1  "<FRS_P1_28_Obj_YPos_Stdev>"
  Data Type Conversion15/1 -> Bus Creator/16
  Bus Selector/1 -> Data Type Conversion/1  "<FRS_P1_28_Msg_CheckSum>"
  Bus Selector/15 -> Data Type Conversion14/1  "<FRS_P2_28_Obj_MeasFlag>"
  Bus Selector/3 -> Data Type Conversion2/1  "<FRS_P1_28_Obj_ExstProb>"
  Bus Selector/13 -> Data Type Conversion12/1  "<FRS_P2_28_Msg_CheckSum>"
  Bus Selector/2 -> Data Type Conversion1/1  "<FRS_P1_28_Msg_AliveCounter>"
  Data Type Conversion11/1 -> Bus Creator/12
  Data Type Conversion5/1 -> Bus Creator/6
  Bus Selector/4 -> Data Type Conversion3/1  "<FRS_P1_28_Obj_XVelRel_Stdev>"
  Bus Selector/7 -> Data Type Conversion6/1  "<FRS_P1_28_Obj_MotionPattern>"
  Data Type Conversion9/1 -> Bus Creator/10
  Bus Selector/6 -> Data Type Conversion5/1  "<FRS_P1_28_Obj_ObstacleProb>"
  Data Type Conversion18/1 -> Bus Creator/19
  Bus Selector/11 -> Data Type Conversion10/1  "<FRS_P1_28_Obj_UpdateFlag>"
  Data Type Conversion17/1 -> Bus Creator/18
  Bus Selector/16 -> Data Type Conversion15/1  "<FRS_P2_28_Obj_YVelRel>"
  Data Type Conversion6/1 -> Bus Creator/7
  Bus Selector/12 -> Data Type Conversion11/1  "<FRS_P1_28_Obj_ID>"
  Data Type Conversion16/1 -> Bus Creator/17
  Bus Selector/9 -> Data Type Conversion8/1  "<FRS_P1_28_Obj_ValidFlag>"
  Bus Selector/17 -> Data Type Conversion16/1  "<FRS_P2_28_Obj_Type>"
  Bus Selector/10 -> Data Type Conversion9/1  "<FRS_P1_28_Obj_XPos_Stdev>"
  Data Type Conversion10/1 -> Bus Creator/11
  Bus Selector/14 -> Data Type Conversion13/1  "<FRS_P2_28_Msg_AliveCounter>"
  Bus Selector/19 -> Data Type Conversion18/1  "<FRS_P2_28_Obj_YPos>"
  Bus Selector/18 -> Data Type Conversion17/1  "<FRS_P2_28_Obj_XPos>"
  Bus Selector/20 -> Data Type Conversion19/1  "<FRS_P2_28_Obj_XVelRel>"
  In1/1 -> Bus Selector/1
  Bus Creator/1 -> Out1/1
  Data Type Conversion/1 -> Bus Creator/1
  Data Type Conversion2/1 -> Bus Creator/3
  Data Type Conversion13/1 -> Bus Creator/14
  Data Type Conversion1/1 -> Bus Creator/2
  Data Type Conversion4/1 -> Bus Creator/5
  Data Type Conversion3/1 -> Bus Creator/4
  Data Type Conversion7/1 -> Bus Creator/8
  Data Type Conversion8/1 -> Bus Creator/9
  Data Type Conversion14/1 -> Bus Creator/15
  Data Type Conversion19/1 -> Bus Creator/20

== system Intergration_simu/Radar410_RX/Subsystem41/Subsystem31 ==
  In1 : Inport
  Bus Creator : BusCreator  Inputs=20  OutDataTypeStr=Bus: Obj_Data  NonVirtualBus=on
      settings: InheritFromInputs=off
  Bus Selector : BusSelector  OutputSignals=FRS_P1_29_Msg_CheckSum,FRS_P1_29_Msg_AliveCounter,FRS_P1_29_Obj_ExstProb,FRS_P1_29_Obj_XVelRel_Stdev,FRS_P1_29_Obj_XAccRel,FRS_P1_29_Obj_ObstacleProb,FRS_P1_29_Obj_MotionPattern,FRS_P1_29_Obj_YPos_Stdev,FRS_P1_29_Obj_ValidFlag,FRS_P1_29_Obj_XPos_Stdev,FRS_P1_29_Obj_UpdateFlag,FRS_P1_29_Obj_ID,FRS_P2_29_Msg_CheckSum,FRS_P2_29_Msg_AliveCounter,FRS_P2_29_Obj_MeasFlag,FRS_P2_29_Obj_YVelRel,FRS_P2_29_Obj_Type,FRS_P2_29_Obj_XPos,FRS_P2_29_Obj_YPos,FRS_P2_29_Obj_XVelRel
  Data Type Conversion{,1..19} (20 alike) : DataTypeConversion  OutDataTypeStr=single
  Out1 : Outport  OutDataTypeStr=Bus: Obj_Data
  wires:
  Data Type Conversion19/1 -> Bus Creator/20
  Data Type Conversion14/1 -> Bus Creator/15
  Data Type Conversion8/1 -> Bus Creator/9
  Data Type Conversion7/1 -> Bus Creator/8
  Data Type Conversion3/1 -> Bus Creator/4
  Data Type Conversion4/1 -> Bus Creator/5
  Data Type Conversion1/1 -> Bus Creator/2
  Data Type Conversion13/1 -> Bus Creator/14
  Data Type Conversion2/1 -> Bus Creator/3
  Data Type Conversion/1 -> Bus Creator/1
  Bus Creator/1 -> Out1/1
  In1/1 -> Bus Selector/1
  Bus Selector/20 -> Data Type Conversion19/1  "<FRS_P2_29_Obj_XVelRel>"
  Bus Selector/18 -> Data Type Conversion17/1  "<FRS_P2_29_Obj_XPos>"
  Bus Selector/19 -> Data Type Conversion18/1  "<FRS_P2_29_Obj_YPos>"
  Bus Selector/14 -> Data Type Conversion13/1  "<FRS_P2_29_Msg_AliveCounter>"
  Data Type Conversion10/1 -> Bus Creator/11
  Bus Selector/10 -> Data Type Conversion9/1  "<FRS_P1_29_Obj_XPos_Stdev>"
  Bus Selector/17 -> Data Type Conversion16/1  "<FRS_P2_29_Obj_Type>"
  Bus Selector/9 -> Data Type Conversion8/1  "<FRS_P1_29_Obj_ValidFlag>"
  Data Type Conversion16/1 -> Bus Creator/17
  Bus Selector/12 -> Data Type Conversion11/1  "<FRS_P1_29_Obj_ID>"
  Data Type Conversion6/1 -> Bus Creator/7
  Bus Selector/16 -> Data Type Conversion15/1  "<FRS_P2_29_Obj_YVelRel>"
  Data Type Conversion17/1 -> Bus Creator/18
  Bus Selector/11 -> Data Type Conversion10/1  "<FRS_P1_29_Obj_UpdateFlag>"
  Data Type Conversion18/1 -> Bus Creator/19
  Bus Selector/6 -> Data Type Conversion5/1  "<FRS_P1_29_Obj_ObstacleProb>"
  Data Type Conversion9/1 -> Bus Creator/10
  Bus Selector/7 -> Data Type Conversion6/1  "<FRS_P1_29_Obj_MotionPattern>"
  Bus Selector/4 -> Data Type Conversion3/1  "<FRS_P1_29_Obj_XVelRel_Stdev>"
  Data Type Conversion5/1 -> Bus Creator/6
  Data Type Conversion11/1 -> Bus Creator/12
  Bus Selector/2 -> Data Type Conversion1/1  "<FRS_P1_29_Msg_AliveCounter>"
  Bus Selector/13 -> Data Type Conversion12/1  "<FRS_P2_29_Msg_CheckSum>"
  Bus Selector/3 -> Data Type Conversion2/1  "<FRS_P1_29_Obj_ExstProb>"
  Bus Selector/15 -> Data Type Conversion14/1  "<FRS_P2_29_Obj_MeasFlag>"
  Bus Selector/1 -> Data Type Conversion/1  "<FRS_P1_29_Msg_CheckSum>"
  Data Type Conversion15/1 -> Bus Creator/16
  Bus Selector/8 -> Data Type Conversion7/1  "<FRS_P1_29_Obj_YPos_Stdev>"
  Bus Selector/5 -> Data Type Conversion4/1  "<FRS_P1_29_Obj_XAccRel>"
  Data Type Conversion12/1 -> Bus Creator/13

== system Intergration_simu/Radar410_RX/Subsystem41/Subsystem32 ==
  In1 : Inport
  Bus Creator : BusCreator  Inputs=20  OutDataTypeStr=Bus: Obj_Data  NonVirtualBus=on
      settings: InheritFromInputs=off
  Bus Selector : BusSelector  OutputSignals=FRS_P1_30_Msg_CheckSum,FRS_P1_30_Msg_AliveCounter,FRS_P1_30_Obj_ExstProb,FRS_P1_30_Obj_XVelRel_Stdev,FRS_P1_30_Obj_XAccRel,FRS_P1_30_Obj_ObstacleProb,FRS_P1_30_Obj_MotionPattern,FRS_P1_30_Obj_YPos_Stdev,FRS_P1_30_Obj_ValidFlag,FRS_P1_30_Obj_XPos_Stdev,FRS_P1_30_Obj_UpdateFlag,FRS_P1_30_Obj_ID,FRS_P2_30_Msg_CheckSum,FRS_P2_30_Msg_AliveCounter,FRS_P2_30_Obj_MeasFlag,FRS_P2_30_Obj_YVelRel,FRS_P2_30_Obj_Type,FRS_P2_30_Obj_XPos,FRS_P2_30_Obj_YPos,FRS_P2_30_Obj_XVelRel
  Data Type Conversion{,1..19} (20 alike) : DataTypeConversion  OutDataTypeStr=single
  Out1 : Outport  OutDataTypeStr=Bus: Obj_Data
  wires:
  Data Type Conversion19/1 -> Bus Creator/20
  Data Type Conversion14/1 -> Bus Creator/15
  Data Type Conversion8/1 -> Bus Creator/9
  Data Type Conversion7/1 -> Bus Creator/8
  Data Type Conversion3/1 -> Bus Creator/4
  Data Type Conversion4/1 -> Bus Creator/5
  Data Type Conversion1/1 -> Bus Creator/2
  Data Type Conversion13/1 -> Bus Creator/14
  Data Type Conversion2/1 -> Bus Creator/3
  Data Type Conversion/1 -> Bus Creator/1
  Bus Creator/1 -> Out1/1
  In1/1 -> Bus Selector/1
  Bus Selector/20 -> Data Type Conversion19/1  "<FRS_P2_30_Obj_XVelRel>"
  Bus Selector/18 -> Data Type Conversion17/1  "<FRS_P2_30_Obj_XPos>"
  Bus Selector/19 -> Data Type Conversion18/1  "<FRS_P2_30_Obj_YPos>"
  Bus Selector/14 -> Data Type Conversion13/1  "<FRS_P2_30_Msg_AliveCounter>"
  Data Type Conversion10/1 -> Bus Creator/11
  Bus Selector/10 -> Data Type Conversion9/1  "<FRS_P1_30_Obj_XPos_Stdev>"
  Bus Selector/17 -> Data Type Conversion16/1  "<FRS_P2_30_Obj_Type>"
  Bus Selector/9 -> Data Type Conversion8/1  "<FRS_P1_30_Obj_ValidFlag>"
  Data Type Conversion16/1 -> Bus Creator/17
  Bus Selector/12 -> Data Type Conversion11/1  "<FRS_P1_30_Obj_ID>"
  Data Type Conversion6/1 -> Bus Creator/7
  Bus Selector/16 -> Data Type Conversion15/1  "<FRS_P2_30_Obj_YVelRel>"
  Data Type Conversion17/1 -> Bus Creator/18
  Bus Selector/11 -> Data Type Conversion10/1  "<FRS_P1_30_Obj_UpdateFlag>"
  Data Type Conversion18/1 -> Bus Creator/19
  Bus Selector/6 -> Data Type Conversion5/1  "<FRS_P1_30_Obj_ObstacleProb>"
  Data Type Conversion9/1 -> Bus Creator/10
  Bus Selector/7 -> Data Type Conversion6/1  "<FRS_P1_30_Obj_MotionPattern>"
  Bus Selector/4 -> Data Type Conversion3/1  "<FRS_P1_30_Obj_XVelRel_Stdev>"
  Data Type Conversion5/1 -> Bus Creator/6
  Data Type Conversion11/1 -> Bus Creator/12
  Bus Selector/2 -> Data Type Conversion1/1  "<FRS_P1_30_Msg_AliveCounter>"
  Bus Selector/13 -> Data Type Conversion12/1  "<FRS_P2_30_Msg_CheckSum>"
  Bus Selector/3 -> Data Type Conversion2/1  "<FRS_P1_30_Obj_ExstProb>"
  Bus Selector/15 -> Data Type Conversion14/1  "<FRS_P2_30_Obj_MeasFlag>"
  Bus Selector/1 -> Data Type Conversion/1  "<FRS_P1_30_Msg_CheckSum>"
  Data Type Conversion15/1 -> Bus Creator/16
  Bus Selector/8 -> Data Type Conversion7/1  "<FRS_P1_30_Obj_YPos_Stdev>"
  Bus Selector/5 -> Data Type Conversion4/1  "<FRS_P1_30_Obj_XAccRel>"
  Data Type Conversion12/1 -> Bus Creator/13

== system Intergration_simu/Radar410_RX/Subsystem41/Subsystem33 ==
  In1 : Inport
  Bus Creator : BusCreator  Inputs=20  OutDataTypeStr=Bus: Obj_Data  NonVirtualBus=on
      settings: InheritFromInputs=off
  Bus Selector : BusSelector  OutputSignals=FRS_P1_31_Msg_CheckSum,FRS_P1_31_Msg_AliveCounter,FRS_P1_31_Obj_ExstProb,FRS_P1_31_Obj_XVelRel_Stdev,FRS_P1_31_Obj_XAccRel,FRS_P1_31_Obj_ObstacleProb,FRS_P1_31_Obj_MotionPattern,FRS_P1_31_Obj_YPos_Stdev,FRS_P1_31_Obj_ValidFlag,FRS_P1_31_Obj_XPos_Stdev,FRS_P1_31_Obj_UpdateFlag,FRS_P1_31_Obj_ID,FRS_P2_31_Msg_CheckSum,FRS_P2_31_Msg_AliveCounter,FRS_P2_31_Obj_MeasFlag,FRS_P2_31_Obj_YVelRel,FRS_P2_31_Obj_Type,FRS_P2_31_Obj_XPos,FRS_P2_31_Obj_YPos,FRS_P2_31_Obj_XVelRel
  Data Type Conversion{,1..19} (20 alike) : DataTypeConversion  OutDataTypeStr=single
  Out1 : Outport  OutDataTypeStr=Bus: Obj_Data
  wires:
  Data Type Conversion12/1 -> Bus Creator/13
  Bus Selector/5 -> Data Type Conversion4/1  "<FRS_P1_31_Obj_XAccRel>"
  Bus Selector/8 -> Data Type Conversion7/1  "<FRS_P1_31_Obj_YPos_Stdev>"
  Data Type Conversion15/1 -> Bus Creator/16
  Bus Selector/1 -> Data Type Conversion/1  "<FRS_P1_31_Msg_CheckSum>"
  Bus Selector/15 -> Data Type Conversion14/1  "<FRS_P2_31_Obj_MeasFlag>"
  Bus Selector/3 -> Data Type Conversion2/1  "<FRS_P1_31_Obj_ExstProb>"
  Bus Selector/13 -> Data Type Conversion12/1  "<FRS_P2_31_Msg_CheckSum>"
  Bus Selector/2 -> Data Type Conversion1/1  "<FRS_P1_31_Msg_AliveCounter>"
  Data Type Conversion11/1 -> Bus Creator/12
  Data Type Conversion5/1 -> Bus Creator/6
  Bus Selector/4 -> Data Type Conversion3/1  "<FRS_P1_31_Obj_XVelRel_Stdev>"
  Bus Selector/7 -> Data Type Conversion6/1  "<FRS_P1_31_Obj_MotionPattern>"
  Data Type Conversion9/1 -> Bus Creator/10
  Bus Selector/6 -> Data Type Conversion5/1  "<FRS_P1_31_Obj_ObstacleProb>"
  Data Type Conversion18/1 -> Bus Creator/19
  Bus Selector/11 -> Data Type Conversion10/1  "<FRS_P1_31_Obj_UpdateFlag>"
  Data Type Conversion17/1 -> Bus Creator/18
  Bus Selector/16 -> Data Type Conversion15/1  "<FRS_P2_31_Obj_YVelRel>"
  Data Type Conversion6/1 -> Bus Creator/7
  Bus Selector/12 -> Data Type Conversion11/1  "<FRS_P1_31_Obj_ID>"
  Data Type Conversion16/1 -> Bus Creator/17
  Bus Selector/9 -> Data Type Conversion8/1  "<FRS_P1_31_Obj_ValidFlag>"
  Bus Selector/17 -> Data Type Conversion16/1  "<FRS_P2_31_Obj_Type>"
  Bus Selector/10 -> Data Type Conversion9/1  "<FRS_P1_31_Obj_XPos_Stdev>"
  Data Type Conversion10/1 -> Bus Creator/11
  Bus Selector/14 -> Data Type Conversion13/1  "<FRS_P2_31_Msg_AliveCounter>"
  Bus Selector/19 -> Data Type Conversion18/1  "<FRS_P2_31_Obj_YPos>"
  Bus Selector/18 -> Data Type Conversion17/1  "<FRS_P2_31_Obj_XPos>"
  Bus Selector/20 -> Data Type Conversion19/1  "<FRS_P2_31_Obj_XVelRel>"
  In1/1 -> Bus Selector/1
  Bus Creator/1 -> Out1/1
  Data Type Conversion/1 -> Bus Creator/1
  Data Type Conversion2/1 -> Bus Creator/3
  Data Type Conversion13/1 -> Bus Creator/14
  Data Type Conversion1/1 -> Bus Creator/2
  Data Type Conversion4/1 -> Bus Creator/5
  Data Type Conversion3/1 -> Bus Creator/4
  Data Type Conversion7/1 -> Bus Creator/8
  Data Type Conversion8/1 -> Bus Creator/9
  Data Type Conversion14/1 -> Bus Creator/15
  Data Type Conversion19/1 -> Bus Creator/20

== system Intergration_simu/Radar410_RX/Subsystem41/Subsystem34 ==
  In1 : Inport
  Bus Creator : BusCreator  Inputs=20  OutDataTypeStr=Bus: Obj_Data  NonVirtualBus=on
      settings: InheritFromInputs=off
  Bus Selector : BusSelector  OutputSignals=FRS_P1_32_Msg_CheckSum,FRS_P1_32_Msg_AliveCounter,FRS_P1_32_Obj_ExstProb,FRS_P1_32_Obj_XVelRel_Stdev,FRS_P1_32_Obj_XAccRel,FRS_P1_32_Obj_ObstacleProb,FRS_P1_32_Obj_MotionPattern,FRS_P1_32_Obj_YPos_Stdev,FRS_P1_32_Obj_ValidFlag,FRS_P1_32_Obj_XPos_Stdev,FRS_P1_32_Obj_UpdateFlag,FRS_P1_32_Obj_ID,FRS_P2_32_Msg_CheckSum,FRS_P2_32_Msg_AliveCounter,FRS_P2_32_Obj_MeasFlag,FRS_P2_32_Obj_YVelRel,FRS_P2_32_Obj_Type,FRS_P2_32_Obj_XPos,FRS_P2_32_Obj_YPos,FRS_P2_32_Obj_XVelRel
  Data Type Conversion{,1..19} (20 alike) : DataTypeConversion  OutDataTypeStr=single
  Out1 : Outport  OutDataTypeStr=Bus: Obj_Data
  wires:
  Data Type Conversion12/1 -> Bus Creator/13
  Bus Selector/5 -> Data Type Conversion4/1  "<FRS_P1_32_Obj_XAccRel>"
  Bus Selector/8 -> Data Type Conversion7/1  "<FRS_P1_32_Obj_YPos_Stdev>"
  Data Type Conversion15/1 -> Bus Creator/16
  Bus Selector/1 -> Data Type Conversion/1  "<FRS_P1_32_Msg_CheckSum>"
  Bus Selector/15 -> Data Type Conversion14/1  "<FRS_P2_32_Obj_MeasFlag>"
  Bus Selector/3 -> Data Type Conversion2/1  "<FRS_P1_32_Obj_ExstProb>"
  Bus Selector/13 -> Data Type Conversion12/1  "<FRS_P2_32_Msg_CheckSum>"
  Bus Selector/2 -> Data Type Conversion1/1  "<FRS_P1_32_Msg_AliveCounter>"
  Data Type Conversion11/1 -> Bus Creator/12
  Data Type Conversion5/1 -> Bus Creator/6
  Bus Selector/4 -> Data Type Conversion3/1  "<FRS_P1_32_Obj_XVelRel_Stdev>"
  Bus Selector/7 -> Data Type Conversion6/1  "<FRS_P1_32_Obj_MotionPattern>"
  Data Type Conversion9/1 -> Bus Creator/10
  Bus Selector/6 -> Data Type Conversion5/1  "<FRS_P1_32_Obj_ObstacleProb>"
  Data Type Conversion18/1 -> Bus Creator/19
  Bus Selector/11 -> Data Type Conversion10/1  "<FRS_P1_32_Obj_UpdateFlag>"
  Data Type Conversion17/1 -> Bus Creator/18
  Bus Selector/16 -> Data Type Conversion15/1  "<FRS_P2_32_Obj_YVelRel>"
  Data Type Conversion6/1 -> Bus Creator/7
  Bus Selector/12 -> Data Type Conversion11/1  "<FRS_P1_32_Obj_ID>"
  Data Type Conversion16/1 -> Bus Creator/17
  Bus Selector/9 -> Data Type Conversion8/1  "<FRS_P1_32_Obj_ValidFlag>"
  Bus Selector/17 -> Data Type Conversion16/1  "<FRS_P2_32_Obj_Type>"
  Bus Selector/10 -> Data Type Conversion9/1  "<FRS_P1_32_Obj_XPos_Stdev>"
  Data Type Conversion10/1 -> Bus Creator/11
  Bus Selector/14 -> Data Type Conversion13/1  "<FRS_P2_32_Msg_AliveCounter>"
  Bus Selector/19 -> Data Type Conversion18/1  "<FRS_P2_32_Obj_YPos>"
  Bus Selector/18 -> Data Type Conversion17/1  "<FRS_P2_32_Obj_XPos>"
  Bus Selector/20 -> Data Type Conversion19/1  "<FRS_P2_32_Obj_XVelRel>"
  In1/1 -> Bus Selector/1
  Bus Creator/1 -> Out1/1
  Data Type Conversion/1 -> Bus Creator/1
  Data Type Conversion2/1 -> Bus Creator/3
  Data Type Conversion13/1 -> Bus Creator/14
  Data Type Conversion1/1 -> Bus Creator/2
  Data Type Conversion4/1 -> Bus Creator/5
  Data Type Conversion3/1 -> Bus Creator/4
  Data Type Conversion7/1 -> Bus Creator/8
  Data Type Conversion8/1 -> Bus Creator/9
  Data Type Conversion14/1 -> Bus Creator/15
  Data Type Conversion19/1 -> Bus Creator/20
